simulink model "DisturbanceModels"  (R2023a)
settings: Solver=VariableStepAuto  StartTime=0.0  StopTime=30000  RelTol=1e-8
undefined symbols (not defined in the file or in its folder): A, e_0, eps_Eb, eta_Eb, I, IAU, m, omega_0, orbit, p, rho, rho_a, s_eci
libraries: sharedtransform x4, aerolibtransform2 x3, matrix_library x2, aerolibgravity2 x1
settings Model: Creator=rbrown  LastModifiedBy=Josh2
settings SolverCC: AllowMultiTaskInputOutput=on  ZeroCrossControl=DisableAll
settings DebuggingCC: ReadBeforeWriteMsg=DisableAll  WriteAfterWriteMsg=DisableAll  WriteAfterReadMsg=DisableAll  MultiTaskDSMMsg=none
settings ModelReferenceCC: UpdateModelReferenceTargets=IfOutOfDate

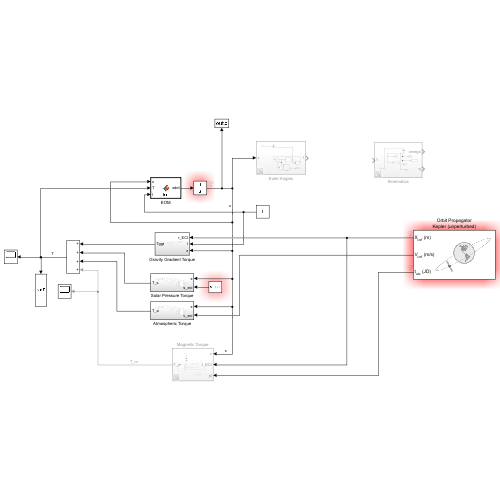
[thumbnail: Simulink's stored preview of the top-level diagram]
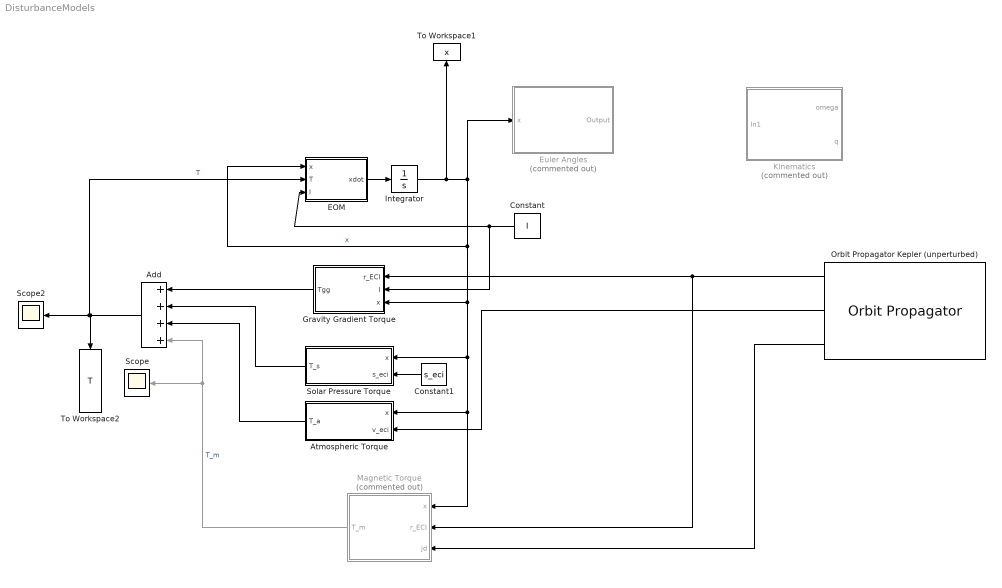
== system DisturbanceModels ==
  Add : Sum  Inputs=++++
  Atmospheric Torque : Subsystem
  Constant : Constant  Value=I
  Constant1 : Constant  Value=s_eci
  EOM : MATLAB Function  TreatAsAtomicUnit=on
  Euler Angles : Subsystem  Commented=on
  Gravity Gradient Torque : Subsystem
  Integrator : Integrator  InitialCondition=[eps_Eb; eta_Eb; omega_0]  AbsoluteTolerance=1e-8
  Kinematics : Subsystem  Commented=on
  Magnetic Torque : Subsystem  Commented=on
  Orbit Propagator Kepler (unperturbed) : OrbitPropagator  startDate=jd_0  action=Error  semiMajorAxis=orbit.a*1e3  eccentricity=orbit.e  inclination=orbit.i  raan=orbit.Omega  argPeriapsis=orbit.AOP  trueAnomaly=orbit.theta  inertialPosition=[3649700.0 3308200.0 -4676600.0]  inertialVelocity=[-2750.8 6666.4 2573.4]  fixedPosition=[-4142689.0 -2676864.7 -4669861.6]  fixedVelocity=[1452.7 -6720.7 2568.1]  customR=3396200  customMu=4.305e13  customJ2=1.0826269e-03  customOmega=4.06125949e-3
  Scope : Scope
  Scope2 : Scope
  Solar Pressure Torque : Subsystem
  To Workspace1 : ToWorkspace  VariableName=x  SampleTime=-1
      settings: Save2DSignal=2-D array (concatenate along first dimension)
  To Workspace2 : ToWorkspace  VariableName=T  SampleTime=-1
      settings: Save2DSignal=2-D array (concatenate along first dimension)
  wires:
  EOM/1(xdot) -> Integrator/1
  Add/1 -> Scope2/1, EOM/2(T), To Workspace2/1  "T"
  Orbit Propagator Kepler (unperturbed)/1 -> Magnetic Torque/2(r_ECI), Gravity Gradient Torque/1(r_ECI)
  Integrator/1 -> To Workspace1/1, Euler Angles/1(x), Atmospheric Torque/1(x), Magnetic Torque/1(x), Solar Pressure Torque/1(x), Gravity Gradient Torque/3(x), EOM/1(x)  "x"
  Constant/1 -> Gravity Gradient Torque/2(I), EOM/3(I)
  Magnetic Torque/1(T_m) -> Add/4, Scope/1  "T_m"
  Orbit Propagator Kepler (unperturbed)/3 -> Magnetic Torque/3(jd)
  Gravity Gradient Torque/1(Tgg) -> Add/1
  Constant1/1 -> Solar Pressure Torque/2(s_eci)
  Solar Pressure Torque/1(T_s) -> Add/2
  Orbit Propagator Kepler (unperturbed)/2 -> Atmospheric Torque/2(v_eci)
  Atmospheric Torque/1(T_a) -> Add/3

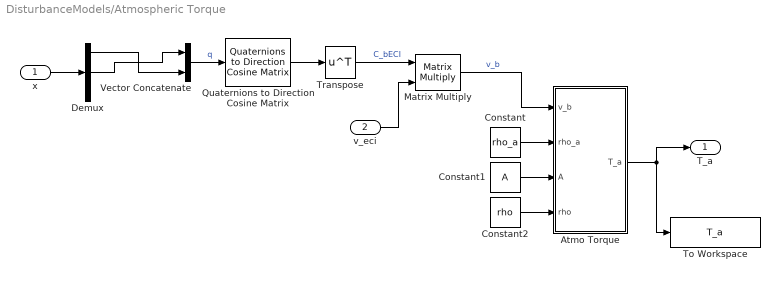
== system DisturbanceModels/Atmospheric Torque ==
  x : Inport
  v_eci : Inport  Port=2
  Atmo Torque : MATLAB Function  TreatAsAtomicUnit=on
  Constant : Constant  Value=rho_a
  Constant1 : Constant  Value=A
  Constant2 : Constant  Value=rho
  Demux : Demux  Outputs=[3, 1, -1]
  Matrix Multiply : Product  Multiplication=Matrix(*)
  Quaternions to Direction Cosine Matrix : sharedtransform/Quaternions to  Direction Cosine Matrix  aMode=aMode
      settings: LibrarySourceBlock=|
      | aerolibtransform2/Quaternions to
      | Direction Cosine Matrix
  To Workspace : ToWorkspace  VariableName=T_a  SampleTime=-1
      settings: Save2DSignal=2-D array (concatenate along first dimension)
  Transpose : Math  Operator=transpose
  Vector Concatenate : Concatenate
  T_a : Outport
  wires:
  Constant/1 -> Atmo Torque/2(rho_a)
  Transpose/1 -> Matrix Multiply/1  "C_bECI"
  Quaternions to Direction Cosine Matrix/1 -> Transpose/1
  Vector Concatenate/1 -> Quaternions to Direction Cosine Matrix/1  "q"
  Demux/1 -> Vector Concatenate/2
  Demux/2 -> Vector Concatenate/1
  x/1 -> Demux/1
  v_eci/1 -> Matrix Multiply/2
  Matrix Multiply/1 -> Atmo Torque/1(v_b)  "v_b"
  Atmo Torque/1(T_a) -> T_a/1, To Workspace/1
  Constant1/1 -> Atmo Torque/3(A)
  Constant2/1 -> Atmo Torque/4(rho)

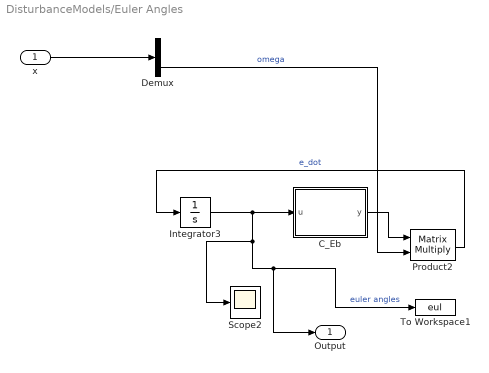
== system DisturbanceModels/Euler Angles ==
  x : Inport
  C_Eb : MATLAB Function  TreatAsAtomicUnit=on
  Demux : Demux  Outputs=[-1, 3]
  Integrator3 : Integrator  InitialCondition=e_0
  Product2 : Product  Multiplication=Matrix(*)
  Scope2 : Scope
  To Workspace1 : ToWorkspace  VariableName=eul  SampleTime=-1
  Output : Outport
  wires:
  Product2/1 -> Integrator3/1  "e_dot"
  C_Eb/1(y) -> Product2/1
  Integrator3/1 -> Output/1, To Workspace1/1, Scope2/1, C_Eb/1(u)  "euler angles"
  x/1 -> Demux/1
  Demux/2 -> Product2/2  "omega"

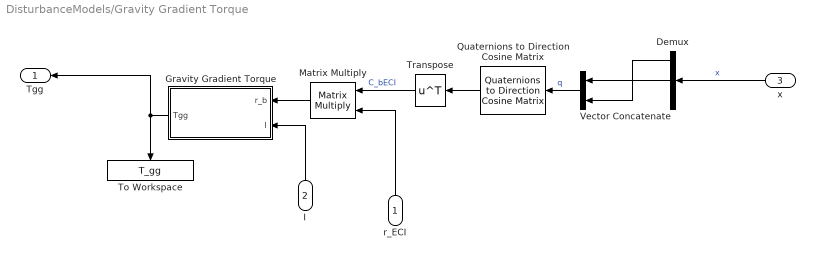
== system DisturbanceModels/Gravity Gradient Torque ==
  r_ECI : Inport
  I : Inport  Port=2
  x : Inport  Port=3
  Demux : Demux  Outputs=[3, 1, -1]
  Gravity Gradient Torque : MATLAB Function  TreatAsAtomicUnit=on
  Matrix Multiply : Product  Multiplication=Matrix(*)
  Quaternions to Direction Cosine Matrix : sharedtransform/Quaternions to  Direction Cosine Matrix  aMode=aMode
      settings: LibrarySourceBlock=|
      | aerolibtransform2/Quaternions to
      | Direction Cosine Matrix
  To Workspace : ToWorkspace  VariableName=T_gg  SampleTime=-1
      settings: Save2DSignal=2-D array (concatenate along first dimension)
  Transpose : Math  Operator=transpose
  Vector Concatenate : Concatenate
  Tgg : Outport
  wires:
  Gravity Gradient Torque/1(Tgg) -> Tgg/1, To Workspace/1
  r_ECI/1 -> Matrix Multiply/2
  I/1 -> Gravity Gradient Torque/2(I)
  x/1 -> Demux/1  "x"
  Vector Concatenate/1 -> Quaternions to Direction Cosine Matrix/1  "q"
  Demux/1 -> Vector Concatenate/2
  Demux/2 -> Vector Concatenate/1
  Matrix Multiply/1 -> Gravity Gradient Torque/1(r_b)
  Quaternions to Direction Cosine Matrix/1 -> Transpose/1
  Transpose/1 -> Matrix Multiply/1  "C_bECI"

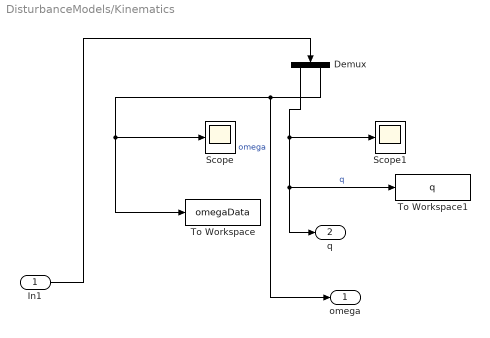
== system DisturbanceModels/Kinematics ==
  In1 : Inport
  Demux : Demux  Outputs=[-1 3]
  Scope : Scope
  Scope1 : Scope
  To Workspace : ToWorkspace  VariableName=omegaData  SampleTime=-1
  To Workspace1 : ToWorkspace  VariableName=q  SampleTime=-1
  omega : Outport
  q : Outport  Port=2
  wires:
  Demux/2 -> omega/1, To Workspace/1, Scope/1  "omega"
  Demux/1 -> q/1, To Workspace1/1, Scope1/1  "q"
  In1/1 -> Demux/1

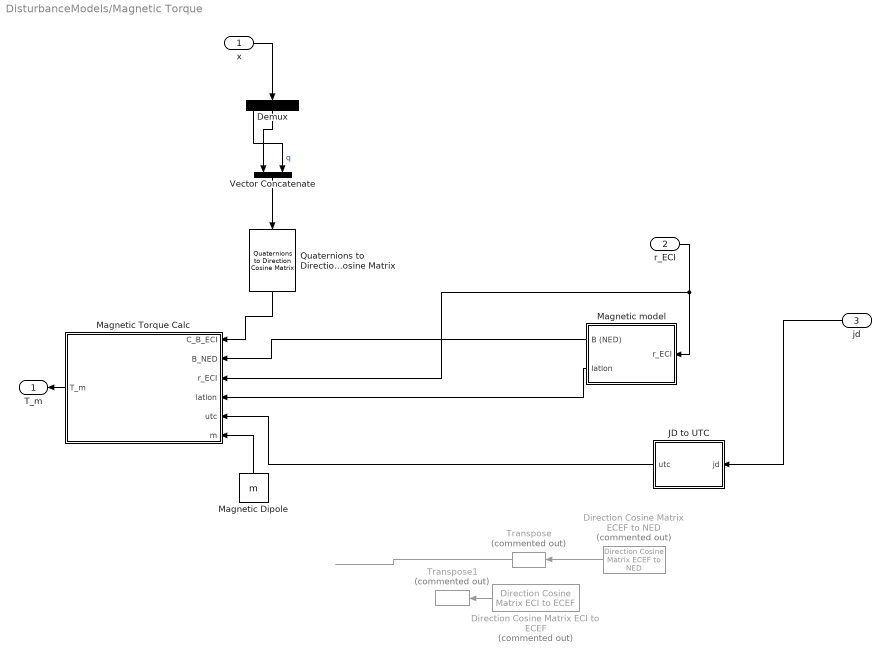
== system DisturbanceModels/Magnetic Torque ==
  x : Inport
  r_ECI : Inport  Port=2
  jd : Inport  Port=3
  Demux : Demux  Outputs=[3 1 -1]
  Direction Cosine Matrix ECEF to NED : aerolibtransform2/Direction Cosine Matrix ECEF to NED  Commented=on
  Direction Cosine Matrix ECI to ECEF : aerolibtransform2/Direction Cosine Matrix ECI to ECEF  Commented=on  red=IAU-2000/2006  year=2020  month=January  day=1  hour=0  min=0  sec=0  deltaT=Sec  errorflag=Error  extraparamflag=off
      settings: AttributesFormatString=%<red>
  JD to UTC : MATLAB Function  TreatAsAtomicUnit=on
  Magnetic Dipole : Constant  Value=m
  Magnetic Torque Calc : MATLAB Function  TreatAsAtomicUnit=on
  Magnetic model : Subsystem
  Quaternions to Direction Cosine Matrix : sharedtransform/Quaternions to  Direction Cosine Matrix  aMode=aMode
      settings: LibrarySourceBlock=|
      | aerolibtransform2/Quaternions to
      | Direction Cosine Matrix
  Transpose : matrix_library/Transpose  Commented=on
  Transpose1 : matrix_library/Transpose  Commented=on
  Vector Concatenate : Concatenate
  T_m : Outport
  wires:
  jd/1 -> JD to UTC/1(jd)
  Magnetic model/1(B (NED)) -> Magnetic Torque Calc/2(B_NED)
  Magnetic Dipole/1 -> Magnetic Torque Calc/6(m)
  Magnetic model/2(latlon) -> Magnetic Torque Calc/4(latlon)
  JD to UTC/1(utc) -> Magnetic Torque Calc/5(utc)
  r_ECI/1 -> Magnetic model/1(r_ECI), Magnetic Torque Calc/3(r_ECI)
  Magnetic Torque Calc/1(T_m) -> T_m/1
  Quaternions to Direction Cosine Matrix/1 -> Magnetic Torque Calc/1(C_B_ECI)
  Vector Concatenate/1 -> Quaternions to Direction Cosine Matrix/1
  x/1 -> Demux/1
  Demux/2 -> Vector Concatenate/1
  Demux/1 -> Vector Concatenate/2  "q"
  Direction Cosine Matrix ECI to ECEF/1 -> Transpose1/1
  Direction Cosine Matrix ECEF to NED/1 -> Transpose/1
  ? -> Direction Cosine Matrix ECI to ECEF/1
  Transpose/1 -> ?

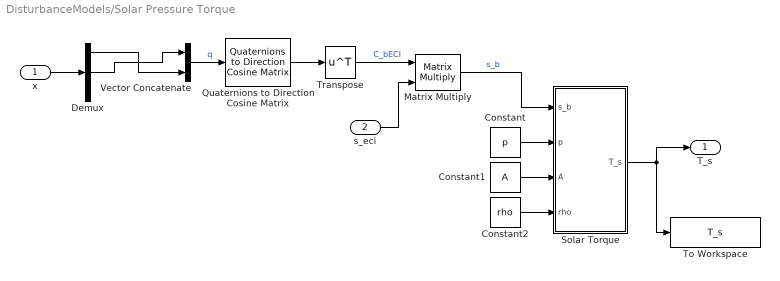
== system DisturbanceModels/Solar Pressure Torque ==
  x : Inport
  s_eci : Inport  Port=2
  Constant : Constant  Value=p
  Constant1 : Constant  Value=A
  Constant2 : Constant  Value=rho
  Demux : Demux  Outputs=[3, 1, -1]
  Matrix Multiply : Product  Multiplication=Matrix(*)
  Quaternions to Direction Cosine Matrix : sharedtransform/Quaternions to  Direction Cosine Matrix  aMode=aMode
      settings: LibrarySourceBlock=|
      | aerolibtransform2/Quaternions to
      | Direction Cosine Matrix
  Solar Torque : MATLAB Function  TreatAsAtomicUnit=on
  To Workspace : ToWorkspace  VariableName=T_s  SampleTime=-1
      settings: Save2DSignal=2-D array (concatenate along first dimension)
  Transpose : Math  Operator=transpose
  Vector Concatenate : Concatenate
  T_s : Outport
  wires:
  Constant/1 -> Solar Torque/2(p)
  Transpose/1 -> Matrix Multiply/1  "C_bECI"
  Quaternions to Direction Cosine Matrix/1 -> Transpose/1
  Vector Concatenate/1 -> Quaternions to Direction Cosine Matrix/1  "q"
  Demux/1 -> Vector Concatenate/2
  Demux/2 -> Vector Concatenate/1
  x/1 -> Demux/1
  s_eci/1 -> Matrix Multiply/2
  Matrix Multiply/1 -> Solar Torque/1(s_b)  "s_b"
  Solar Torque/1(T_s) -> T_s/1, To Workspace/1
  Constant1/1 -> Solar Torque/3(A)
  Constant2/1 -> Solar Torque/4(rho)

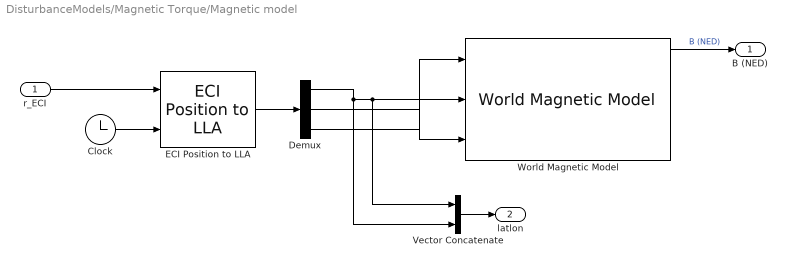
== system DisturbanceModels/Magnetic Torque/Magnetic model ==
  r_ECI : Inport
  Clock : Clock
  Demux : Demux  Outputs=3
  ECI Position to LLA : aerolibtransform2/ECI Position to LLA  red=IAU-2000/2006  year=2013  month=January  day=1  hour=0  min=0  sec=0  deltaT=Sec  errorflag=Error  extraparamflag=off  eunits=Metric (MKS)  earthmodel=WGS84  flat=1/298.257223563  eqradius=6378137
      settings: AttributesFormatString=%<red>
  Vector Concatenate : Concatenate
  World Magnetic Model : aerolibgravity2/World Magnetic Model  model=Custom  customFile='WMM2020.COF'  units=Metric (MKS)  time_in=off  month=January  day=1  year=2020  action=Error  h_out=on  dec_out=on  inc_out=on  ti_out=on
  B (NED) : Outport
  latlon : Outport  Port=2
  wires:
  r_ECI/1 -> ECI Position to LLA/1
  ECI Position to LLA/1 -> Demux/1
  Demux/3 -> World Magnetic Model/1
  Demux/1 -> Vector Concatenate/2, Vector Concatenate/1, World Magnetic Model/2
  Demux/2 -> World Magnetic Model/3
  World Magnetic Model/1 -> B (NED)/1  "B (NED)"
  Vector Concatenate/1 -> latlon/1
  Clock/1 -> ECI Position to LLA/2

== matlab function DisturbanceModels/EOM ==
  data: x input; T input; xdot output; I input
function xdot = fcn(x, T, I)

xdot = zeros(7,1);
eps = x(1:3); 
eta = x(4);
omega = x(5:7);
xdot(1:3) = .5 * (eta *eye(3) + joshCross(eps)) * omega;
xdot(4) = -.5 * eps' * omega;
xdot(5:7) = I^-1 * (-joshCross(omega)*I*omega + T);

end

== matlab function DisturbanceModels/Euler Angles/C_Eb ==
  data: u input; y output
function y = fcn(u)

y = C_e(u);

== matlab function DisturbanceModels/Gravity Gradient Torque/Gravity Gradient Torque ==
  data: Tgg output; r_b input; I input
function Tgg = GG(r_b, I)

mu = 3.986e14; %m 
Tgg = ((3*mu)/norm(r_b)^5)  *joshCross(r_b)*I*r_b;

== matlab function DisturbanceModels/Solar Pressure Torque/Solar Torque ==
  data: s_b input; T_s output; p input; A input; rho input
function T_s = fcn(s_b, p, A, rho)

n = [[1; 0; 0 ], [0; 1; 0], [0; 0; 1], [-1; 0; 0 ], [0; -1; 0], [0; 0; -1]]; %normal vecs
Cp = wettedcenter(s_b, A, n, rho);
Fs = solarforce(s_b, A, n, p);
T_s = cross(Cp, Fs);

end

== matlab function DisturbanceModels/Magnetic Torque/Magnetic Torque Calc ==
  data: C_B_ECI input; B_NED input; r_ECI input; latlon input; utc input; T_m output; m input
function T_m = fcn(C_B_ECI, B_NED, r_ECI, latlon, utc, m)

 


B_b = C_B_ECI * C_ECI_ECEF * C_ECEF_NED * B_NED;

T_m = cross(m, B_b);

== matlab function DisturbanceModels/Magnetic Torque/JD to UTC ==
  data: jd input; utc output
function utc = fcn(jd)

utc = datevec(datetime(jd, "ConvertFrom","juliandate"));

== matlab function DisturbanceModels/Atmospheric Torque/Atmo Torque ==
  data: v_b input; T_a output; rho_a input; A input; rho input
function T_a = fcn(v_b, rho_a, A, rho)

n = [[1; 0; 0 ], [0; 1; 0], [0; 0; 1], [-1; 0; 0 ], [0; -1; 0], [0; 0; -1]]; %normal vecs
Cp = wettedcenter(v_b, A, n, rho);
F_a = aeroforce(v_b, A, n, rho_a);
T_a = cross(Cp, F_a)

end
